simulink library "HDL_ieee_8021513"  (R2024a)
settings: Solver=FixedStepDiscrete  StartTime=0.0  StopTime=10.0  RelTol=1e-3
undefined symbols (not defined in the file): Add, axiWidth, CONST, fs, peakDetectorThreshold, peakDetectorWindow, QAM, Shift
libraries: hdlsllib x199, $bdroot x91, whdlutilities x34, whdledac x9, simulink x8, whdlmod x6, dspsigops x5, dsphdlfiltering2 x4, embreciprocals x3, dsphdlsigops2 x2, commhdlcrc x2, dspstat3 x2
(part 2 of 6)

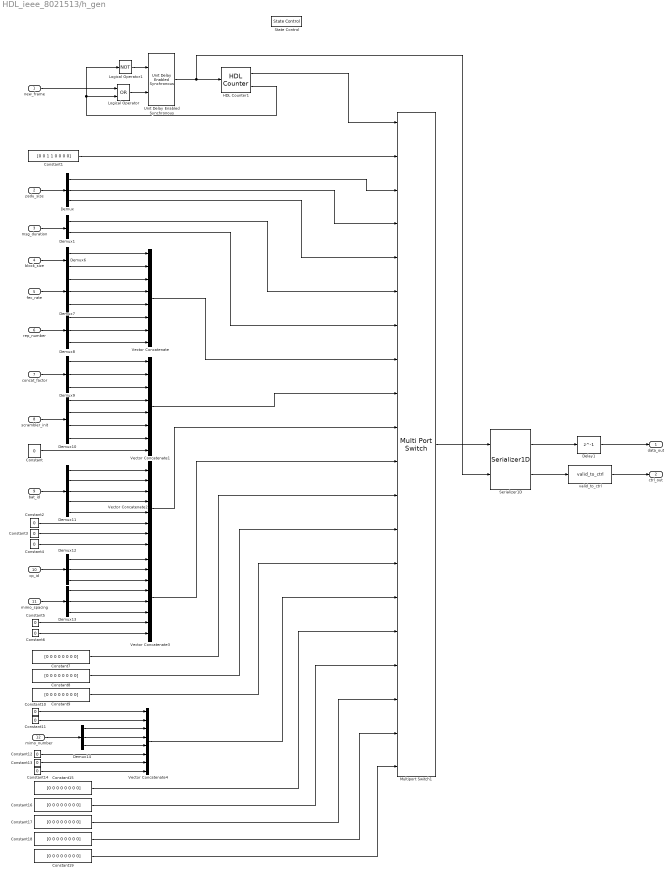
== system HDL_ieee_8021513/h_gen ==
  new_frame : Inport
  psdu_size : Inport  Port=2
  msg_duration : Inport  Port=3
  block_size : Inport  Port=4
  fec_rate : Inport  Port=5
  rep_number : Inport  Port=6
  concat_factor : Inport  Port=7
  scrambler_init : Inport  Port=8
  bat_id : Inport  Port=9
  cp_id : Inport  Port=10
  mimo_spacing : Inport  Port=11
  mimo_number : Inport  Port=12
  Constant{,2..6,10..14} (11 alike) : Constant  Value=0  OutDataTypeStr=boolean  SampleTime=-1
  Constant1 : Constant  Value=[0 0 1 1 0 0 0 0]  VectorParams1D=off  OutDataTypeStr=boolean  SampleTime=-1
  Constant{7..9,15..19} (8 alike) : Constant  Value=[0 0 0 0 0 0 0 0]  VectorParams1D=off  OutDataTypeStr=boolean  SampleTime=-1
  Delay1 : Delay  DelayLength=1  InitialCondition=0  UseCircularBuffer=on
  Demux{,7..9,12..14} (7 alike) : Demux  Outputs=3
  Demux1 : Demux  Outputs=2
  Demux10 : Demux
  Demux11 : Demux  Outputs=5
  Demux6 : Demux  Outputs=2
  HDL Counter1 : hdlsllib/Sources/HDL Counter  CountType=Count limited  CountInit=0  CountStep=1  CountMax=18  CountFromType=Initial value  CountFrom=0  CountResetPort=off  CountLoadPort=off  CountEnbPort=on  CountDirPort=off  CountHitOutputPort=on  CountDataType=Unsigned  CountWordLen=5  CountFracLen=0  CountSampTime=1
  Logical Operator : Logic  Operator=OR  IconShape=distinctive  AllPortsSameDT=off  OutDataTypeStr=boolean
  Logical Operator1 : Logic  Operator=NOT  IconShape=distinctive  AllPortsSameDT=off  OutDataTypeStr=boolean
  Multiport Switch1 : MultiPortSwitch  DataPortOrder=Zero-based contiguous  Inputs=19  zeroidx=on  OutDataTypeStr=Inherit: Same as first data input  SaturateOnIntegerOverflow=off
  Serializer1D : hdlsllib/HDL Operations/Serializer1D  Ratio=8  IdleCycles=0  validIn=on  startOut=off  validOut=on  inputDataDimensions=-1  inputSampleTime=-1  inputSignalType=auto
  State Control : StateControl  StateControl=Synchronous
  Unit Delay Enabled Synchronous : hdlsllib/Discrete/Unit Delay Enabled Synchronous  InitialCondition=0.0  SampleTime=-1
  Vector Concatenate{,1..4} (5 alike) : Concatenate  NumInputs=8  Mode=Multidimensional array  ConcatenateDimension=2
  valid_to_ctrl : $bdroot/valid_to_ctrl  SystemSampleTime=-1  VariantActivationTime=update diagram  AllowFlexibleInterface=on  Latency=0  AutoFrameSizeCalculation=off
  data_out : Outport  VectorParamsAs1DForOutWhenUnconnected=off
  ctrl_out : Outport  Port=2  VectorParamsAs1DForOutWhenUnconnected=off
  wires:
  mimo_number/1 -> Demux14/1
  msg_duration/1 -> Demux1/1
  rep_number/1 -> Demux8/1
  fec_rate/1 -> Demux7/1
  block_size/1 -> Demux6/1
  concat_factor/1 -> Demux9/1
  scrambler_init/1 -> Demux10/1
  Demux/2 -> Multiport Switch1/4
  Demux/3 -> Multiport Switch1/5
  Demux1/2 -> Multiport Switch1/7
  Constant1/1 -> Multiport Switch1/2
  Vector Concatenate/1 -> Multiport Switch1/8
  Constant/1 -> Vector Concatenate1/8
  bat_id/1 -> Demux11/1
  Constant2/1 -> Vector Concatenate2/6
  Constant3/1 -> Vector Concatenate2/7
  Constant4/1 -> Vector Concatenate2/8
  Constant5/1 -> Vector Concatenate3/7
  Constant6/1 -> Vector Concatenate3/8
  Constant10/1 -> Vector Concatenate4/1
  Constant11/1 -> Vector Concatenate4/2
  Constant12/1 -> Vector Concatenate4/6
  Constant13/1 -> Vector Concatenate4/7
  Constant14/1 -> Vector Concatenate4/8
  Vector Concatenate1/1 -> Multiport Switch1/9
  Vector Concatenate2/1 -> Multiport Switch1/10
  Vector Concatenate3/1 -> Multiport Switch1/11
  Constant7/1 -> Multiport Switch1/12
  Constant8/1 -> Multiport Switch1/13
  Constant9/1 -> Multiport Switch1/14
  Vector Concatenate4/1 -> Multiport Switch1/15
  Constant15/1 -> Multiport Switch1/16
  Constant16/1 -> Multiport Switch1/17
  Constant17/1 -> Multiport Switch1/18
  Constant18/1 -> Multiport Switch1/19
  Constant19/1 -> Multiport Switch1/20
  HDL Counter1/1 -> Multiport Switch1/1
  Multiport Switch1/1 -> Serializer1D/1
  Serializer1D/1 -> Delay1/1
  new_frame/1 -> Logical Operator/1
  HDL Counter1/2 -> Logical Operator/2, Logical Operator1/1
  Logical Operator/1 -> Unit Delay Enabled Synchronous/2
  Unit Delay Enabled Synchronous/1 -> Serializer1D/2, HDL Counter1/1
  Logical Operator1/1 -> Unit Delay Enabled Synchronous/1
  Delay1/1 -> data_out/1
  Serializer1D/2 -> valid_to_ctrl/1
  valid_to_ctrl/1 -> ctrl_out/1
  Demux6/1 -> Vector Concatenate/1
  Demux6/2 -> Vector Concatenate/2
  Demux7/1 -> Vector Concatenate/3
  Demux7/2 -> Vector Concatenate/4
  Demux7/3 -> Vector Concatenate/5
  Demux8/1 -> Vector Concatenate/6
  Demux8/2 -> Vector Concatenate/7
  Demux8/3 -> Vector Concatenate/8
  Demux9/1 -> Vector Concatenate1/1
  Demux9/2 -> Vector Concatenate1/2
  Demux9/3 -> Vector Concatenate1/3
  Demux10/1 -> Vector Concatenate1/4
  Demux10/2 -> Vector Concatenate1/5
  Demux10/3 -> Vector Concatenate1/6
  Demux10/4 -> Vector Concatenate1/7
  Demux11/1 -> Vector Concatenate2/1
  Demux11/2 -> Vector Concatenate2/2
  Demux11/3 -> Vector Concatenate2/3
  Demux11/4 -> Vector Concatenate2/4
  Demux11/5 -> Vector Concatenate2/5
  Demux12/1 -> Vector Concatenate3/1
  Demux12/2 -> Vector Concatenate3/2
  Demux12/3 -> Vector Concatenate3/3
  Demux13/1 -> Vector Concatenate3/4
  Demux13/2 -> Vector Concatenate3/5
  Demux13/3 -> Vector Concatenate3/6
  Demux14/1 -> Vector Concatenate4/3
  Demux14/2 -> Vector Concatenate4/4
  Demux14/3 -> Vector Concatenate4/5
  psdu_size/1 -> Demux/1
  cp_id/1 -> Demux12/1
  mimo_spacing/1 -> Demux13/1
  Demux/1 -> Multiport Switch1/3
  Demux1/1 -> Multiport Switch1/6

== system HDL_ieee_8021513/h_remove_repetition ==
  data_in : Inport
  start_in : Inport  Port=2
  HDL Counter : hdlsllib/Sources/HDL Counter  CountType=Count limited  CountInit=0  CountStep=1  CountMax=CONST.headerBitsPerFec-1  CountFromType=Initial value  CountFrom=0  CountResetPort=on  CountLoadPort=off  CountEnbPort=on  CountDirPort=off  CountHitOutputPort=on  CountDataType=Unsigned  CountWordLen=nextpow2(CONST.headerBitsPerFec)  CountFracLen=0  CountSampTime=1
  Logical Operator : Logic  Operator=OR  AllPortsSameDT=off  OutDataTypeStr=boolean
  Sample Control Bus Creator : whdlutilities/Sample Control Bus Creator
  State Control : StateControl  StateControl=Synchronous
  Switch : Switch  Criteria=u2 ~= 0  SaturateOnIntegerOverflow=off  InputSameDT=off
  Terminator : Terminator
  Unit Delay{,1..7} (8 alike) : UnitDelay  SampleTime=-1  HasFrameUpgradeWarning=on
  data_out : Outport
  ctrl_out : Outport  Port=2
  wires:
  Unit Delay7/1 -> Sample Control Bus Creator/3
  Unit Delay6/1 -> Sample Control Bus Creator/1
  Unit Delay5/1 -> data_out/1
  Switch/1 -> Unit Delay/1, HDL Counter/2, Unit Delay7/1
  Unit Delay3/1 -> HDL Counter/1, Unit Delay6/1  "rst"
  Unit Delay4/1 -> Unit Delay5/1  "data_in"
  Unit Delay2/1 -> Switch/1
  Unit Delay1/1 -> Switch/2
  Logical Operator/1 -> Unit Delay1/1
  HDL Counter/1 -> Terminator/1  "count"
  Unit Delay/1 -> Switch/3
  Sample Control Bus Creator/1 -> ctrl_out/1
  data_in/1 -> Unit Delay4/1
  HDL Counter/2 -> Sample Control Bus Creator/2, Logical Operator/2
  start_in/1 -> Unit Delay2/1, Logical Operator/1, Unit Delay3/1

== system HDL_ieee_8021513/h_repetition ==
  data_in : Inport
  ctrl_in : Inport  Port=2
  Bus Selector : BusSelector  OutputSignals=start,end,valid
  Delay{,1..4} (5 alike) : Delay  DelayLength=1  InitialCondition=0  UseCircularBuffer=on
  HDL Counter2 : hdlsllib/Sources/HDL Counter  CountType=Count limited  CountInit=CONST.headerBitsPerFec-2  CountStep=1  CountMax=CONST.headerBitsPerFec-1  CountFromType=Specify  CountFrom=0  CountResetPort=off  CountLoadPort=off  CountEnbPort=on  CountDirPort=off  CountHitOutputPort=off  CountDataType=Unsigned  CountWordLen=nextpow2(CONST.headerBitsPerOFDMSymbol)  CountFracLen=0  CountSampTime=1
  HDL Counter3 : hdlsllib/Sources/HDL Counter  CountType=Count limited  CountInit=0  CountStep=1  CountMax=CONST.headerBitsPerOFDMSymbol - CONST.headerBitsPerFec -1  CountFromType=Initial value  CountFrom=0  CountResetPort=off  CountLoadPort=off  CountEnbPort=on  CountDirPort=off  CountHitOutputPort=on  CountDataType=Unsigned  CountWordLen=nextpow2(CONST.headerBitsPerOFDMSymbol)  CountFracLen=0  CountSampTime=1
  Logical Operator : Logic  Operator=NOT  IconShape=distinctive  AllPortsSameDT=off  OutDataTypeStr=boolean
  Logical Operator1 : Logic  Operator=OR  IconShape=distinctive  AllPortsSameDT=off  OutDataTypeStr=boolean
  Logical Operator2 : Logic  Operator=NOT  IconShape=distinctive  AllPortsSameDT=off  OutDataTypeStr=boolean
  NOT : Logic  Operator=NOT  IconShape=distinctive  AllPortsSameDT=off  OutDataTypeStr=boolean
  Sample Control Bus Creator : whdlutilities/Sample Control Bus Creator
  Simple Dual Port RAM : hdlsllib/HDL RAMs/Simple Dual Port RAM  ram_size=nextpow2(CONST.headerBitsPerOFDMSymbol)
  State Control : StateControl  StateControl=Synchronous
  Switch : Switch  Criteria=u2 ~= 0  SaturateOnIntegerOverflow=off  InputSameDT=off
  Switch1 : Switch  Criteria=u2 ~= 0  SaturateOnIntegerOverflow=off  InputSameDT=off
  Unit Delay Enabled Synchronous1 : hdlsllib/Discrete/Unit Delay Enabled Synchronous  InitialCondition=0.0  SampleTime=-1
  data_out : Outport  VectorParamsAs1DForOutWhenUnconnected=off
  ctrl_out : Outport  Port=2  VectorParamsAs1DForOutWhenUnconnected=off
  wires:
  Delay4/1 -> [end_out]
  Delay3/1 -> Switch1/1
  ctrl_in/1 -> Bus Selector/1
  Bus Selector/3 -> [valid], Delay3/1  "<valid>"
  Sample Control Bus Creator/1 -> ctrl_out/1
  Bus Selector/1 -> Delay/1  "<start>"
  Bus Selector/2 -> [end]  "<end>"
  Delay/1 -> Sample Control Bus Creator/1
  [end_out] -> Sample Control Bus Creator/2
  Switch1/1 -> Sample Control Bus Creator/3
  [valid] -> HDL Counter2/1  "addrB_valid"
  [valid] -> Simple Dual Port RAM/3
  HDL Counter2/1 -> Simple Dual Port RAM/2
  data_in/1 -> Delay1/1, Simple Dual Port RAM/1  "datain"
  HDL Counter3/1 -> Simple Dual Port RAM/4  "addrA"
  Unit Delay Enabled Synchronous1/1 -> HDL Counter3/1, Delay2/1
  [end] -> Logical Operator1/1
  Logical Operator1/1 -> Unit Delay Enabled Synchronous1/2
  HDL Counter3/2 -> Logical Operator1/2, NOT/1, Delay4/1
  NOT/1 -> Unit Delay Enabled Synchronous1/1
  Switch/1 -> data_out/1
  Delay2/1 -> Logical Operator2/1, Switch1/3, Logical Operator/1
  Simple Dual Port RAM/1 -> Switch/3
  Delay1/1 -> Switch/1
  Logical Operator/1 -> Switch1/2
  Logical Operator2/1 -> Switch/2

== system HDL_ieee_8021513/h_rx_full ==
  data_in : Inport
  start_in : Inport  Port=2
  ldpc_in : Inport  Port=3
  ldpc_ctrl_in : Inport  Port=4
  Delay{2..5} (4 alike) : Delay  DelayLength=1  InitialCondition=0  UseCircularBuffer=on
  Rate Transition : RateTransition  OutPortSampleTimeOpt=Multiple of input port sample time  OutPortSampleTimeMultiple=8
  State Control : StateControl  StateControl=Synchronous
  h_crc_rx : $bdroot/h_crc_rx  SystemSampleTime=-1  VariantActivationTime=update diagram  AllowFlexibleInterface=on  Latency=0  AutoFrameSizeCalculation=off
  h_remove_repetition : $bdroot/h_remove_repetition  SystemSampleTime=-1  VariantActivationTime=update diagram  AllowFlexibleInterface=on  Latency=0  AutoFrameSizeCalculation=off
  h_scrambler : $bdroot/h_scrambler  SystemSampleTime=-1  VariantActivationTime=update diagram  AllowFlexibleInterface=on  Latency=0  AutoFrameSizeCalculation=off
      settings: LibrarySourceBlock=|
      | hdlsllib/Ports &
      | Subsystems/Subsystem
  h_separate : $bdroot/h_separate  SystemSampleTime=-1  VariantActivationTime=update diagram  AllowFlexibleInterface=on  Latency=0  AutoFrameSizeCalculation=off
  psdu_size : Outport
  msg_duration : Outport  Port=2
  block_size : Outport  Port=3
  fec_rate : Outport  Port=4
  rep_number : Outport  Port=5
  concat_factor : Outport  Port=6
  scrambler_init : Outport  Port=7
  bat_id : Outport  Port=8
  cp_id : Outport  Port=9
  mimo_spacing : Outport  Port=10
  mimo_number : Outport  Port=11
  end : Outport  Port=12
  err : Outport  Port=13
  ldpc_out : Outport  Port=14  VectorParamsAs1DForOutWhenUnconnected=off
  ldpc_ctrl_out : Outport  Port=15  VectorParamsAs1DForOutWhenUnconnected=off
  wires:
  Delay5/1 -> end/1
  Delay4/1 -> err/1
  Delay3/1 -> h_scrambler/2
  Delay2/1 -> h_scrambler/1
  h_remove_repetition/1 -> ldpc_out/1
  h_remove_repetition/2 -> ldpc_ctrl_out/1
  Rate Transition/1 -> Delay4/1
  h_separate/4 -> fec_rate/1
  h_separate/1 -> psdu_size/1
  ldpc_ctrl_in/1 -> Delay3/1
  h_crc_rx/2 -> h_separate/2
  h_scrambler/2 -> h_crc_rx/2
  h_separate/7 -> scrambler_init/1
  h_scrambler/1 -> h_crc_rx/1
  h_separate/5 -> rep_number/1
  h_separate/11 -> mimo_number/1
  h_crc_rx/1 -> h_separate/1
  h_separate/9 -> cp_id/1
  h_crc_rx/3 -> Rate Transition/1
  ldpc_in/1 -> Delay2/1
  h_separate/8 -> bat_id/1
  h_separate/2 -> msg_duration/1
  h_separate/10 -> mimo_spacing/1
  h_separate/6 -> concat_factor/1
  h_separate/12 -> Delay5/1
  h_separate/3 -> block_size/1
  data_in/1 -> h_remove_repetition/1
  start_in/1 -> h_remove_repetition/2

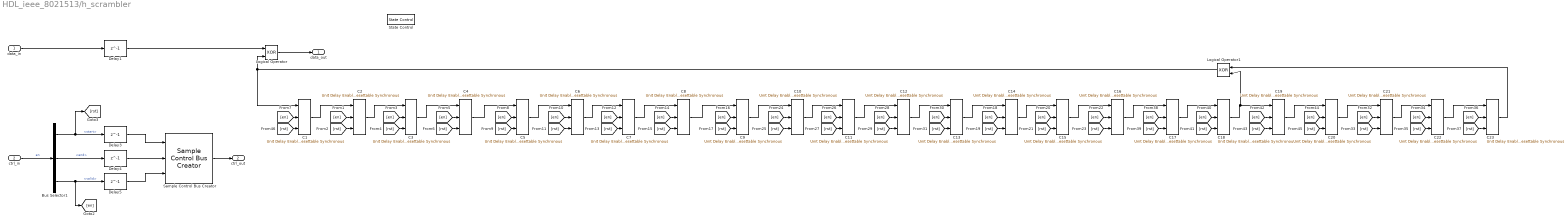
== system HDL_ieee_8021513/h_scrambler ==
  data_in : Inport
  ctrl_in : Inport  Port=2
  Bus Selector1 : BusSelector  OutputSignals=start,end,valid
  C{1,3,5,7,9,11,13,15,17,19,21,23} (12 alike) : hdlsllib/Discrete/Unit Delay Enabled Resettable Synchronous  InitialCondition=0  SampleTime=-1
  C{2,4,6,8,10,12,14,16,18,20,22} (11 alike) : hdlsllib/Discrete/Unit Delay Enabled Resettable Synchronous  InitialCondition=1  SampleTime=-1
  Delay{1,3..5} (4 alike) : Delay  DelayLength=1  InitialCondition=0  UseCircularBuffer=on
  Logical Operator : Logic  Operator=XOR  IconShape=distinctive  AllPortsSameDT=off  OutDataTypeStr=boolean
  Logical Operator1 : Logic  Operator=XOR  IconShape=distinctive  AllPortsSameDT=off  OutDataTypeStr=boolean
  Sample Control Bus Creator : whdlutilities/Sample Control Bus Creator
  State Control : StateControl  StateControl=Synchronous
  data_out : Outport
  ctrl_out : Outport  Port=2  VectorParamsAs1DForOutWhenUnconnected=off
  wires:
  Sample Control Bus Creator/1 -> ctrl_out/1
  Delay5/1 -> Sample Control Bus Creator/3
  Delay4/1 -> Sample Control Bus Creator/2
  Delay3/1 -> Sample Control Bus Creator/1
  Bus Selector1/3 -> Delay5/1, [en]  "<valid>"
  Bus Selector1/2 -> Delay4/1  "<end>"
  Bus Selector1/1 -> Delay3/1, [rst]  "<start>"
  C23/1 -> Logical Operator1/1
  [rst] -> C22/3
  C19/1 -> C20/1
  [en] -> C20/2
  [en] -> C21/2
  C21/1 -> C22/1
  [rst] -> C18/3
  [en] -> C17/2
  [rst] -> C19/3
  [rst] -> C21/3
  C17/1 -> C18/1
  C22/1 -> C23/1
  [en] -> C19/2
  [en] -> C18/2
  [en] -> C23/2
  [rst] -> C20/3
  [en] -> C22/2
  C16/1 -> C17/1
  [rst] -> C23/3
  [rst] -> C17/3
  C8/1 -> C9/1
  [rst] -> C15/3
  [en] -> C15/2
  [en] -> C14/2
  [rst] -> C16/3
  [en] -> C12/2
  [rst] -> C14/3
  C13/1 -> C14/1
  C11/1 -> C12/1
  [rst] -> C9/3
  [en] -> C10/2
  [en] -> C9/2
  C14/1 -> C15/1
  [en] -> C11/2
  [rst] -> C13/3
  C10/1 -> C11/1
  [rst] -> C10/3
  C12/1 -> C13/1
  [en] -> C13/2
  [rst] -> C11/3
  [en] -> C16/2
  [rst] -> C12/3
  C9/1 -> C10/1
  C15/1 -> C16/1
  [rst] -> C5/3
  [en] -> C6/2
  C6/1 -> C7/1
  [en] -> C8/2
  [rst] -> C6/3
  C5/1 -> C6/1
  [rst] -> C7/3
  C7/1 -> C8/1
  [rst] -> C8/3
  [en] -> C7/2
  [en] -> C5/2
  Delay1/1 -> Logical Operator/1
  data_in/1 -> Delay1/1
  ctrl_in/1 -> Bus Selector1/1  "en"
  Logical Operator/1 -> data_out/1
  [rst] -> C3/3
  [en] -> C3/2
  Logical Operator1/1 -> Logical Operator/2, C1/1
  [rst] -> C2/3
  C1/1 -> C2/1
  C3/1 -> C4/1
  [en] -> C1/2
  [rst] -> C1/3
  C4/1 -> C5/1
  [en] -> C4/2
  C2/1 -> C3/1
  [rst] -> C4/3
  [en] -> C2/2
  C20/1 -> C21/1
  C18/1 -> Logical Operator1/2, C19/1

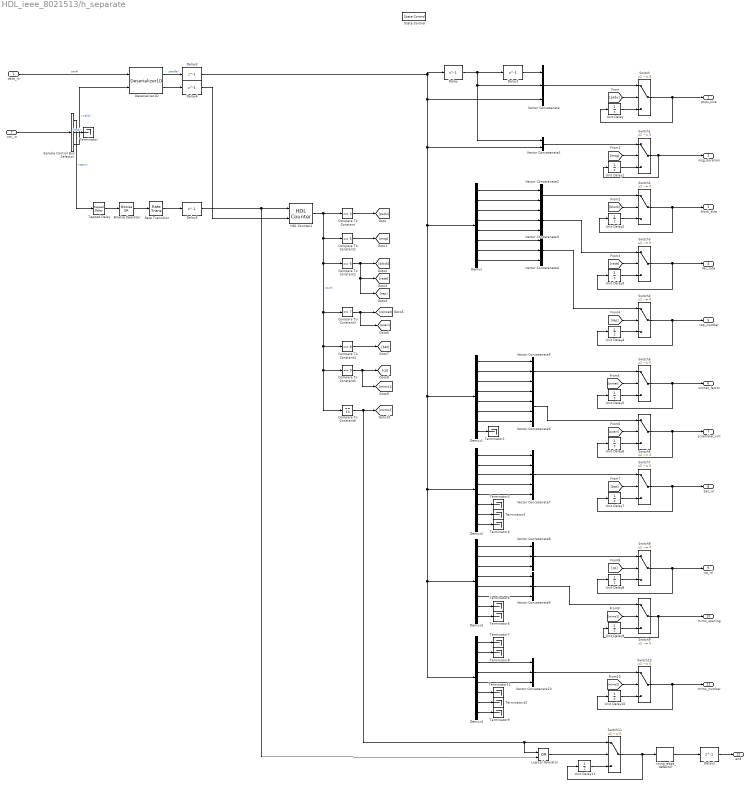
== system HDL_ieee_8021513/h_separate ==
  data_in : Inport
  ctrl_in : Inport  Port=2
  Bitwise Operator : simulink/Logic and Bit Operations/Bitwise Operator  logicop=OR  UseBitMask=off  BitMask=bin2dec('11011001')  BitMaskRealWorld=Stored Integer
      settings: LibrarySourceBlock=|
      | hdlsllib/Logic and Bit
      | Operations/Bitwise
      | Operator
  Compare To Constant : hdlsllib/Logic and Bit Operations/Compare To Constant  relop===  const=3  OutDataTypeStr=boolean
  Compare To Constant1 : hdlsllib/Logic and Bit Operations/Compare To Constant  relop===  const=5  OutDataTypeStr=boolean
  Compare To Constant2 : hdlsllib/Logic and Bit Operations/Compare To Constant  relop===  const=6  OutDataTypeStr=boolean
  Compare To Constant3 : hdlsllib/Logic and Bit Operations/Compare To Constant  relop===  const=7  OutDataTypeStr=boolean
  Compare To Constant4 : hdlsllib/Logic and Bit Operations/Compare To Constant  relop===  const=8  OutDataTypeStr=boolean
  Compare To Constant5 : hdlsllib/Logic and Bit Operations/Compare To Constant  relop===  const=9  OutDataTypeStr=boolean
  Compare To Constant6 : hdlsllib/Logic and Bit Operations/Compare To Constant  relop===  const=13  OutDataTypeStr=boolean
  Delay{,1..5} (6 alike) : Delay  DelayLength=1  InitialCondition=0  UseCircularBuffer=on
  Demux{,1..4} (5 alike) : Demux  Outputs=8
  Deserializer1D : hdlsllib/HDL Operations/Deserializer1D  Ratio=8  IdleCycles=0  InitialCondition=0  startIn=off  validIn=on  validOut=on  inputDataDimensions=-1  inputSampleTime=-1  inputSignalType=auto
  HDL Counter1 : hdlsllib/Sources/HDL Counter  CountType=Free running  CountInit=0  CountStep=1  CountMax=25  CountFromType=Initial value  CountFrom=0  CountResetPort=on  CountLoadPort=off  CountEnbPort=on  CountDirPort=off  CountHitOutputPort=off  CountDataType=Unsigned  CountWordLen=5  CountFracLen=0  CountSampTime=1
  Logical Operator : Logic  Operator=OR  IconShape=distinctive  AllPortsSameDT=off  OutDataTypeStr=boolean
  Rate Transition : RateTransition  OutPortSampleTimeOpt=Multiple of input port sample time  OutPortSampleTimeMultiple=8
  Sample Control Bus Selector : whdlutilities/Sample Control Bus Selector  OutputSignals=start,end,valid
  State Control : StateControl  StateControl=Synchronous
  Switch{,1..11} (12 alike) : Switch  Criteria=u2 ~= 0  SaturateOnIntegerOverflow=off  InputSameDT=off
  Tapped Delay : simulink/Discrete/Tapped Delay  vinit=0.0  samptime=-1  NumDelays=8  DelayOrder=Oldest  includeCurrent=off
      settings: LibrarySourceBlock=hdlsllib/Discrete/Tapped Delay
  Terminator{,1..11} (12 alike) : Terminator
  Unit Delay{,1..11} (12 alike) : UnitDelay  SampleTime=-1  HasFrameUpgradeWarning=on
  Vector Concatenate{,3..5,8..10} (7 alike) : Concatenate  NumInputs=3
  Vector Concatenate1 : Concatenate
  Vector Concatenate2 : Concatenate
  Vector Concatenate6 : Concatenate  NumInputs=4
  Vector Concatenate7 : Concatenate  NumInputs=5
  rising_edge_detector : $bdroot/rising_edge_detector  SystemSampleTime=-1  VariantActivationTime=update diagram  AllowFlexibleInterface=on  Latency=0  AutoFrameSizeCalculation=off
  psdu_size : Outport
  msg_duration : Outport  Port=2
  block_size : Outport  Port=3
  fec_rate : Outport  Port=4
  rep_number : Outport  Port=5
  concat_factor : Outport  Port=6
  scrambler_init : Outport  Port=7
  bat_id : Outport  Port=8
  cp_id : Outport  Port=9
  mimo_spacing : Outport  Port=10
  mimo_number : Outport  Port=11
  end : Outport  Port=12  VectorParamsAs1DForOutWhenUnconnected=off
  wires:
  Delay5/1 -> HDL Counter1/1, Logical Operator/2
  Delay4/1 -> HDL Counter1/2
  Delay3/1 -> Vector Concatenate/3, Vector Concatenate1/2, Demux/1, Demux1/1, Demux2/1, Demux3/1, Demux4/1, Delay/1
  rising_edge_detector/1 -> Delay2/1
  Bitwise Operator/1 -> Rate Transition/1
  Tapped Delay/1 -> Bitwise Operator/1
  Delay2/1 -> end/1
  Logical Operator/1 -> Switch11/2
  Compare To Constant6/1 -> [mimo2], Switch11/1, Logical Operator/1
  Unit Delay11/1 -> Switch11/3
  Switch11/1 -> rising_edge_detector/1, Unit Delay11/1
  Vector Concatenate10/1 -> Switch10/1
  Demux4/5 -> Vector Concatenate10/3
  Demux4/4 -> Vector Concatenate10/2
  Demux4/3 -> Vector Concatenate10/1
  Demux4/6 -> Terminator11/1
  Demux4/7 -> Terminator10/1
  Demux4/8 -> Terminator9/1
  Demux4/2 -> Terminator8/1
  Demux4/1 -> Terminator7/1
  Vector Concatenate9/1 -> Switch9/1
  Vector Concatenate8/1 -> Switch8/1
  Demux3/3 -> Vector Concatenate8/3
  Demux3/2 -> Vector Concatenate8/2
  Demux3/1 -> Vector Concatenate8/1
  Demux3/6 -> Vector Concatenate9/3
  Demux3/5 -> Vector Concatenate9/2
  Demux3/4 -> Vector Concatenate9/1
  Demux3/7 -> Terminator6/1
  Demux3/8 -> Terminator5/1
  Vector Concatenate7/1 -> Switch7/1
  Demux2/5 -> Vector Concatenate7/5
  Demux2/4 -> Vector Concatenate7/4
  Demux2/3 -> Vector Concatenate7/3
  Demux2/2 -> Vector Concatenate7/2
  Demux2/1 -> Vector Concatenate7/1
  Demux2/8 -> Terminator4/1
  Demux2/7 -> Terminator3/1
  Demux2/6 -> Terminator2/1
  Vector Concatenate6/1 -> Switch6/1
  Demux1/8 -> Terminator1/1
  Demux1/7 -> Vector Concatenate6/4
  Demux1/6 -> Vector Concatenate6/3
  Demux1/5 -> Vector Concatenate6/2
  Demux1/4 -> Vector Concatenate6/1
  Vector Concatenate5/1 -> Switch5/1
  Demux1/3 -> Vector Concatenate5/3
  Demux1/2 -> Vector Concatenate5/2
  Demux1/1 -> Vector Concatenate5/1
  Vector Concatenate4/1 -> Switch4/1
  Demux/8 -> Vector Concatenate4/3
  Demux/7 -> Vector Concatenate4/2
  Demux/6 -> Vector Concatenate4/1
  Vector Concatenate3/1 -> Switch3/1
  Demux/5 -> Vector Concatenate3/3
  Demux/4 -> Vector Concatenate3/2
  Demux/3 -> Vector Concatenate3/1
  Vector Concatenate2/1 -> Switch2/1
  Demux/2 -> Vector Concatenate2/2
  Demux/1 -> Vector Concatenate2/1
  Sample Control Bus Selector/2 -> Terminator/1  "<end>"
  Vector Concatenate1/1 -> Switch1/1
  [mimo2] -> Switch10/2
  Switch10/1 -> Unit Delay10/1, mimo_number/1
  Unit Delay10/1 -> Switch10/3
  [mimo1] -> Switch9/2
  Switch9/1 -> Unit Delay9/1, mimo_spacing/1
  Unit Delay9/1 -> Switch9/3
  [cp] -> Switch8/2
  Switch8/1 -> Unit Delay8/1, cp_id/1
  Unit Delay8/1 -> Switch8/3
  [bat] -> Switch7/2
  Switch7/1 -> Unit Delay7/1, bat_id/1
  Unit Delay7/1 -> Switch7/3
  [scram] -> Switch6/2
  Switch6/1 -> Unit Delay6/1, scrambler_init/1
  Unit Delay6/1 -> Switch6/3
  [concat] -> Switch5/2
  Switch5/1 -> Unit Delay5/1, concat_factor/1
  Unit Delay5/1 -> Switch5/3
  [rep] -> Switch4/2
  Switch4/1 -> Unit Delay4/1, rep_number/1
  Unit Delay4/1 -> Switch4/3
  [rate] -> Switch3/2
  Switch3/1 -> Unit Delay3/1, fec_rate/1
  Unit Delay3/1 -> Switch3/3
  [block] -> Switch2/2
  Switch2/1 -> Unit Delay2/1, block_size/1
  Unit Delay2/1 -> Switch2/3
  Switch1/1 -> Unit Delay1/1, msg_duration/1
  Unit Delay1/1 -> Switch1/3
  [msg] -> Switch1/2
  [psdu] -> Switch/2
  Compare To Constant5/1 -> [cp], [mimo1]
  Compare To Constant4/1 -> [bat]
  Compare To Constant3/1 -> [concat], [scram]
  Compare To Constant2/1 -> [rep], [rate], [block]
  Compare To Constant1/1 -> [msg]
  Compare To Constant/1 -> [psdu]
  HDL Counter1/1 -> Compare To Constant/1, Compare To Constant1/1, Compare To Constant2/1, Compare To Constant3/1, Compare To Constant4/1, Compare To Constant5/1, Compare To Constant6/1  "count"
  Rate Transition/1 -> Delay5/1
  Deserializer1D/2 -> Delay4/1
  Unit Delay/1 -> Switch/3
  Switch/1 -> psdu_size/1, Unit Delay/1
  Vector Concatenate/1 -> Switch/1
  Delay1/1 -> Vector Concatenate/1
  Delay/1 -> Delay1/1, Vector Concatenate/2, Vector Concatenate1/1
  Deserializer1D/1 -> Delay3/1  "parallel"
  data_in/1 -> Deserializer1D/1  "serial"
  Sample Control Bus Selector/1 -> Tapped Delay/1  "<start>"
  Sample Control Bus Selector/3 -> Deserializer1D/2  "<valid>"
  ctrl_in/1 -> Sample Control Bus Selector/1

== system HDL_ieee_8021513/header_fec ==
  data_in : Inport
  ctrl_in : Inport  Port=2
  Delay{,1..3} (4 alike) : Delay  DelayLength=1  InitialCondition=0  UseCircularBuffer=on
  Hc_12H_B14 : whdledac/LDPC Encoder  ParityCheckMatrix=CONST.Hc_12H  BlockSize=14  SimulateUsing=Code generation
  State Control : StateControl  StateControl=Synchronous
  Terminator : Terminator
  data_out : Outport
  ctrl_out : Outport  Port=2
  wires:
  Delay3/1 -> Hc_12H_B14/1
  Delay2/1 -> Hc_12H_B14/2
  Delay1/1 -> data_out/1
  Delay/1 -> ctrl_out/1
  ctrl_in/1 -> Delay2/1
  data_in/1 -> Delay3/1
  Hc_12H_B14/2 -> Delay/1
  Hc_12H_B14/1 -> Delay1/1
  Hc_12H_B14/3 -> Terminator/1

== system HDL_ieee_8021513/header_full ==
  new_frame : Inport
  psdu_size : Inport  Port=2
  msg_duration : Inport  Port=3
  block_size : Inport  Port=4
  fec_rate : Inport  Port=5
  rep_number : Inport  Port=6
  concat_factor : Inport  Port=7
  scrambler_init : Inport  Port=8
  bat_id : Inport  Port=9
  cp_id : Inport  Port=10
  mimo_spacing : Inport  Port=11
  mimo_number : Inport  Port=12
  State Control : StateControl  StateControl=Synchronous
  h_crc : $bdroot/h_crc  SystemSampleTime=-1  VariantActivationTime=update diagram  AllowFlexibleInterface=on  Latency=0  AutoFrameSizeCalculation=off
  h_gen : $bdroot/h_gen  SystemSampleTime=-1  VariantActivationTime=update diagram  AllowFlexibleInterface=on  Latency=0  AutoFrameSizeCalculation=off
  h_repetition : $bdroot/h_repetition  SystemSampleTime=-1  VariantActivationTime=update diagram  AllowFlexibleInterface=on  Latency=0  AutoFrameSizeCalculation=off
  h_scrambler : $bdroot/h_scrambler  SystemSampleTime=-1  VariantActivationTime=update diagram  AllowFlexibleInterface=on  Latency=0  AutoFrameSizeCalculation=off
      settings: LibrarySourceBlock=|
      | hdlsllib/Ports &
      | Subsystems/Subsystem
  header_fec : $bdroot/header_fec  SystemSampleTime=-1  VariantActivationTime=update diagram  AllowFlexibleInterface=on  Latency=0  AutoFrameSizeCalculation=off
  header : Outport  VectorParamsAs1DForOutWhenUnconnected=off
  ctrl_out : Outport  Port=2  VectorParamsAs1DForOutWhenUnconnected=off
  wires:
  h_scrambler/1 -> header_fec/1
  h_scrambler/2 -> header_fec/2
  header_fec/1 -> h_repetition/1  "dataOut"
  header_fec/2 -> h_repetition/2
  h_crc/2 -> h_scrambler/2
  h_crc/1 -> h_scrambler/1
  h_gen/2 -> h_crc/2
  h_gen/1 -> h_crc/1
  h_repetition/2 -> ctrl_out/1
  h_repetition/1 -> header/1
  new_frame/1 -> h_gen/1
  psdu_size/1 -> h_gen/2
  msg_duration/1 -> h_gen/3
  block_size/1 -> h_gen/4
  fec_rate/1 -> h_gen/5
  rep_number/1 -> h_gen/6
  concat_factor/1 -> h_gen/7
  scrambler_init/1 -> h_gen/8
  bat_id/1 -> h_gen/9
  cp_id/1 -> h_gen/10
  mimo_spacing/1 -> h_gen/11
  mimo_number/1 -> h_gen/12

== system HDL_ieee_8021513/interpolator ==
  data_in : Inport
  valid_in : Inport  Port=2
  Delay{,4,6..11,14..15,18} (11 alike) : Delay  DelayLength=1  InitialCondition=0  UseCircularBuffer=on
  Delay1 : Delay  DelayLength=CONST.txInterpolatorDelay  InitialCondition=0  UseCircularBuffer=on
  Delay16 : Delay  DelayLength=CONST.txInterpolatorDelay*(CONST.txL-1)  InitialCondition=0  UseCircularBuffer=on
  Delay17 : Delay  DelayLength=CONST.txInterpolatorDelay*(CONST.txL-1)  InitialCondition=0  UseCircularBuffer=on
  Delay2 : Delay  InitialCondition=0  UseCircularBuffer=on
  Delay3 : Delay  DelayLength=CONST.txInterpolatorDelay  InitialCondition=0  UseCircularBuffer=on
  Delay5 : Delay  InitialCondition=0  UseCircularBuffer=on
  FIR Interpolator : dsphdlfiltering2/FIR Interpolator  Numerator=CONST.txInterpolatorFilter.Numerator  FilterStructure=Direct form systolic  InterpolationFactor=CONST.txL  NumCycles=CONST.txL  SimulateUsing=Code generation  roundingMode=Floor  overflowMode=off  CoefficientsDataTypeStr=CONST.txInterpolatorCoefficientsDataType  OutputDataTypeStr=CONST.txInterpolatorOutputDataType  ResetInputPort=off  HDLGlobalReset=on
  HDL Counter : hdlsllib/Sources/HDL Counter  CountType=Count limited  CountInit=0  CountStep=1  CountMax=CONST.txInterpolatorDelay*(CONST.txL-1)-1  CountFromType=Initial value  CountFrom=0  CountResetPort=on  CountLoadPort=off  CountEnbPort=on  CountDirPort=off  CountHitOutputPort=on  CountDataType=Unsigned  CountWordLen=8  CountFracLen=0  CountSampTime=1
  Logical Operator : Logic  Operator=OR  IconShape=distinctive  AllPortsSameDT=off  OutDataTypeStr=boolean
  Logical Operator1 : Logic  IconShape=distinctive  AllPortsSameDT=off  OutDataTypeStr=boolean
  Logical Operator2 : Logic  AllPortsSameDT=off  OutDataTypeStr=boolean
  Logical Operator3 : Logic  Operator=NOT  AllPortsSameDT=off  OutDataTypeStr=boolean
  Logical Operator4 : Logic  Operator=OR  AllPortsSameDT=off  OutDataTypeStr=boolean
  State Control : StateControl  StateControl=Synchronous
  Switch : Switch  Criteria=u2 ~= 0  SaturateOnIntegerOverflow=off  InputSameDT=off
  Terminator : Terminator
  Terminator1 : Terminator
  Unit Delay : UnitDelay  SampleTime=-1  HasFrameUpgradeWarning=on
  Upsample : dspsigops/Upsample  FactorSource=Dialog parameter  N=CONST.txL  Nmax=16  phase=0  RateOptions=Allow multirate processing  ic=0  mode=Unused parameter value
      settings: LibrarySourceBlock=dsphdlsupportsigops/Upsample
  Upsample1 : dspsigops/Upsample  FactorSource=Dialog parameter  N=CONST.txL  Nmax=16  phase=0  RateOptions=Allow multirate processing  ic=0  mode=Unused parameter value
      settings: LibrarySourceBlock=dsphdlsupportsigops/Upsample
  falling_edge_detector : $bdroot/falling_edge_detector  SystemSampleTime=-1  VariantActivationTime=update diagram  AllowFlexibleInterface=on  Latency=0  AutoFrameSizeCalculation=off
  data_out : Outport  VectorParamsAs1DForOutWhenUnconnected=off
  valid_out : Outport  Port=2  VectorParamsAs1DForOutWhenUnconnected=off
  wires:
  Delay18/1 -> Logical Operator3/1
  Logical Operator3/1 -> Logical Operator2/2
  Delay7/1 -> Logical Operator4/2
  Logical Operator4/1 -> Switch/2
  Delay15/1 -> Delay16/1
  Delay14/1 -> Delay15/1
  Delay17/1 -> Delay4/1
  Delay16/1 -> Logical Operator2/1
  Delay10/1 -> HDL Counter/1, Switch/1, Logical Operator4/1
  Switch/1 -> Unit Delay/1, HDL Counter/2, Delay18/1  "count_enable"
  Unit Delay/1 -> Switch/3
  HDL Counter/1 -> Terminator/1  "count"
  HDL Counter/2 -> Delay7/1
  Logical Operator2/1 -> Delay/1
  Delay11/1 -> Delay17/1
  Delay9/1 -> Delay6/1
  Delay8/1 -> Delay14/1, falling_edge_detector/1
  Delay6/1 -> Delay11/1
  falling_edge_detector/1 -> Delay10/1  "b"
  Delay5/1 -> Upsample/1
  Delay2/1 -> Upsample1/1
  data_in/1 -> Delay5/1
  FIR Interpolator/1 -> Delay9/1
  Upsample1/1 -> FIR Interpolator/2
  valid_in/1 -> Delay3/1, Logical Operator/1
  Delay/1 -> valid_out/1
  FIR Interpolator/3 -> Terminator1/1
  Delay1/1 -> Logical Operator1/2
  Delay3/1 -> Logical Operator/2
  Logical Operator/1 -> Delay2/1
  Upsample/1 -> FIR Interpolator/1
  Logical Operator1/1 -> Delay8/1
  Delay4/1 -> data_out/1
  FIR Interpolator/2 -> Delay1/1, Logical Operator1/1

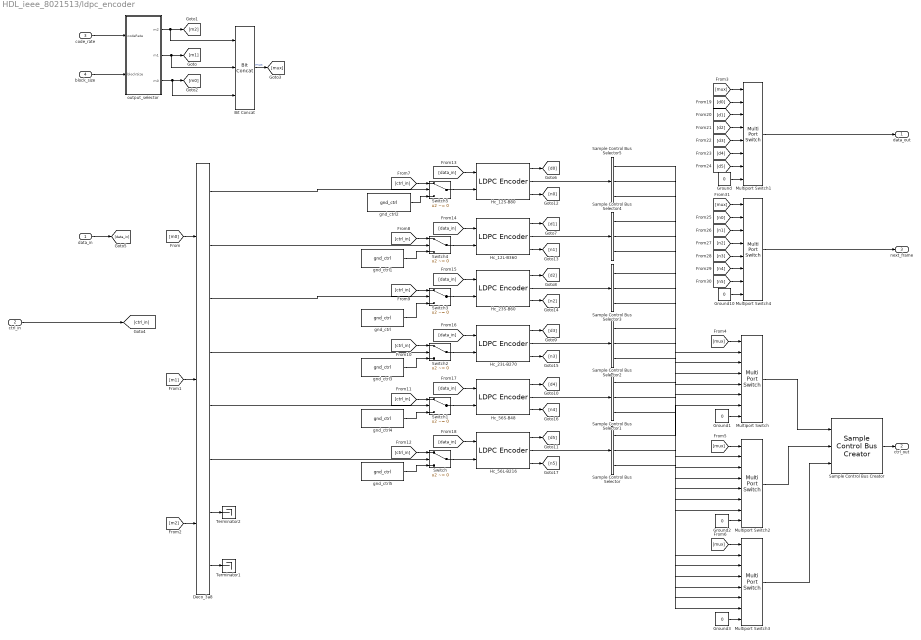
== system HDL_ieee_8021513/ldpc_encoder ==
  data_in : Inport
  ctrl_in : Inport  Port=2
  code_rate : Inport  Port=3
  block_size : Inport  Port=4
  Bit Concat : hdlsllib/Logic and Bit Operations/Bit Concat  numInputs=3
  Deco_3a8 : $bdroot/Deco_3a8  SystemSampleTime=-1  VariantActivationTime=update diagram  AllowFlexibleInterface=on  Latency=0  AutoFrameSizeCalculation=off
  Ground{,1..3,10} (5 alike) : Constant  Value=0  OutDataTypeStr=Inherit: Inherit via back propagation  SampleTime=-1
  Hc_12L-B360 : whdledac/LDPC Encoder  ParityCheckMatrix=CONST.Hc_12L  BlockSize=360  SimulateUsing=Code generation
  Hc_12S-B80 : whdledac/LDPC Encoder  ParityCheckMatrix=CONST.Hc_12S  BlockSize=80  SimulateUsing=Code generation
  Hc_23L-B270 : whdledac/LDPC Encoder  ParityCheckMatrix=CONST.Hc_23L  BlockSize=270  SimulateUsing=Code generation
  Hc_23S-B60 : whdledac/LDPC Encoder  ParityCheckMatrix=CONST.Hc_23S  BlockSize=60  SimulateUsing=Code generation
  Hc_56L-B216 : whdledac/LDPC Encoder  ParityCheckMatrix=CONST.Hc_56L  BlockSize=216  SimulateUsing=Code generation
  Hc_56S-B48 : whdledac/LDPC Encoder  ParityCheckMatrix=CONST.Hc_56S  BlockSize=48  SimulateUsing=Code generation
  Multiport Switch{,1..4} (5 alike) : MultiPortSwitch  DataPortOrder=Zero-based contiguous  Inputs=6  DataPortForDefault=Additional data port  DiagnosticForDefault=None  zeroidx=on  SaturateOnIntegerOverflow=off  InputSameDT=off
  Sample Control Bus Creator : whdlutilities/Sample Control Bus Creator
  Sample Control Bus Selector{,1..5} (6 alike) : whdlutilities/Sample Control Bus Selector  OutputSignals=start,end,valid
  Switch{,1..5} (6 alike) : Switch  Criteria=u2 ~= 0  SaturateOnIntegerOverflow=off  InputSameDT=off  OutDataTypeStr=Inherit: Same as first input
  Terminator1 : Terminator
  Terminator2 : Terminator
  gnd_ctrl{,1..5} (6 alike) : $bdroot/gnd_ctrl  SystemSampleTime=-1  VariantActivationTime=update diagram  AllowFlexibleInterface=on  Latency=0  AutoFrameSizeCalculation=off
  output_selector : Subsystem
  data_out : Outport
  ctrl_out : Outport  Port=2
  next_frame : Outport  Port=3
  wires:
  Multiport Switch1/1 -> data_out/1
  Switch/1 -> Hc_56L-B216/2
  Deco_3a8/8 -> Terminator1/1
  Deco_3a8/7 -> Terminator2/1
  Deco_3a8/6 -> Switch/2
  Switch5/1 -> Hc_12S-B80/2
  Switch4/1 -> Hc_12L-B360/2
  Switch3/1 -> Hc_23S-B60/2
  Switch2/1 -> Hc_23L-B270/2
  Switch1/1 -> Hc_56S-B48/2
  Deco_3a8/1 -> Switch5/2
  Deco_3a8/2 -> Switch4/2
  Deco_3a8/3 -> Switch3/2
  Deco_3a8/4 -> Switch2/2
  Deco_3a8/5 -> Switch1/2
  Hc_12L-B360/3 -> [n1]
  Hc_12S-B80/3 -> [n0]
  Hc_23S-B60/3 -> [n2]
  Hc_23L-B270/3 -> [n3]
  Hc_56S-B48/3 -> [n4]
  Hc_56L-B216/3 -> [n5]
  gnd_ctrl/1 -> Switch3/3
  Hc_56L-B216/2 -> Sample Control Bus Selector/1
  Sample Control Bus Selector/3 -> Multiport Switch3/7
  Sample Control Bus Selector/2 -> Multiport Switch2/7
  Sample Control Bus Selector/1 -> Multiport Switch/7
  Hc_56S-B48/2 -> Sample Control Bus Selector1/1
  Sample Control Bus Selector1/3 -> Multiport Switch3/6
  Sample Control Bus Selector1/2 -> Multiport Switch2/6
  Sample Control Bus Selector1/1 -> Multiport Switch/6
  Hc_23L-B270/2 -> Sample Control Bus Selector2/1
  Sample Control Bus Selector2/3 -> Multiport Switch3/5
  Sample Control Bus Selector2/2 -> Multiport Switch2/5
  Sample Control Bus Selector2/1 -> Multiport Switch/5
  Hc_23S-B60/2 -> Sample Control Bus Selector3/1
  Sample Control Bus Selector3/3 -> Multiport Switch3/4
  Sample Control Bus Selector3/2 -> Multiport Switch2/4
  Sample Control Bus Selector3/1 -> Multiport Switch/4
  Hc_12L-B360/2 -> Sample Control Bus Selector4/1
  Sample Control Bus Selector4/1 -> Multiport Switch/3
  Sample Control Bus Selector4/3 -> Multiport Switch3/3
  Sample Control Bus Selector4/2 -> Multiport Switch2/3
  Hc_12S-B80/2 -> Sample Control Bus Selector5/1
  Sample Control Bus Selector5/3 -> Multiport Switch3/2
  Sample Control Bus Selector5/2 -> Multiport Switch2/2
  Sample Control Bus Selector5/1 -> Multiport Switch/2
  Multiport Switch/1 -> Sample Control Bus Creator/1
  Multiport Switch2/1 -> Sample Control Bus Creator/2
  Multiport Switch3/1 -> Sample Control Bus Creator/3
  Sample Control Bus Creator/1 -> ctrl_out/1
  Ground/1 -> Multiport Switch1/8
  Ground1/1 -> Multiport Switch/8
  Ground2/1 -> Multiport Switch2/8
  Ground3/1 -> Multiport Switch3/8
  code_rate/1 -> output_selector/1(codeRate)
  block_size/1 -> output_selector/2(blockSize)
  output_selector/1(m2) -> Bit Concat/1, [m2]
  output_selector/3(m0) -> Bit Concat/3, [m0]
  output_selector/2(m1) -> Bit Concat/2, [m1]
  Bit Concat/1 -> [mux]  "mux"
  [m0] -> Deco_3a8/1
  [m1] -> Deco_3a8/2
  [m2] -> Deco_3a8/3
  [mux] -> Multiport Switch1/1
  [mux] -> Multiport Switch/1
  [mux] -> Multiport Switch2/1
  [mux] -> Multiport Switch3/1
  [ctrl_in] -> Switch5/1
  [ctrl_in] -> Switch4/1
  [ctrl_in] -> Switch3/1
  [ctrl_in] -> Switch2/1
  [ctrl_in] -> Switch1/1
  [ctrl_in] -> Switch/1
  data_in/1 -> [data_in]
  [data_in] -> Hc_12S-B80/1
  [data_in] -> Hc_12L-B360/1
  [data_in] -> Hc_23S-B60/1
  [data_in] -> Hc_23L-B270/1
  [data_in] -> Hc_56S-B48/1
  [data_in] -> Hc_56L-B216/1
  Hc_12S-B80/1 -> [d0]
  Hc_12L-B360/1 -> [d1]
  Hc_23S-B60/1 -> [d2]
  Hc_23L-B270/1 -> [d3]
  Hc_56S-B48/1 -> [d4]
  Hc_56L-B216/1 -> [d5]
  [d0] -> Multiport Switch1/2
  [d1] -> Multiport Switch1/3
  [d2] -> Multiport Switch1/4
  [d3] -> Multiport Switch1/5
  [d4] -> Multiport Switch1/6
  [d5] -> Multiport Switch1/7
  [n5] -> Multiport Switch4/7
  [n1] -> Multiport Switch4/3
  [n4] -> Multiport Switch4/6
  [n2] -> Multiport Switch4/4
  [mux] -> Multiport Switch4/1
  [n0] -> Multiport Switch4/2
  [n3] -> Multiport Switch4/5
  Multiport Switch4/1 -> next_frame/1
  Ground10/1 -> Multiport Switch4/8
  ctrl_in/1 -> [ctrl_in]
  gnd_ctrl1/1 -> Switch4/3
  gnd_ctrl2/1 -> Switch5/3
  gnd_ctrl3/1 -> Switch2/3
  gnd_ctrl4/1 -> Switch1/3
  gnd_ctrl5/1 -> Switch/3

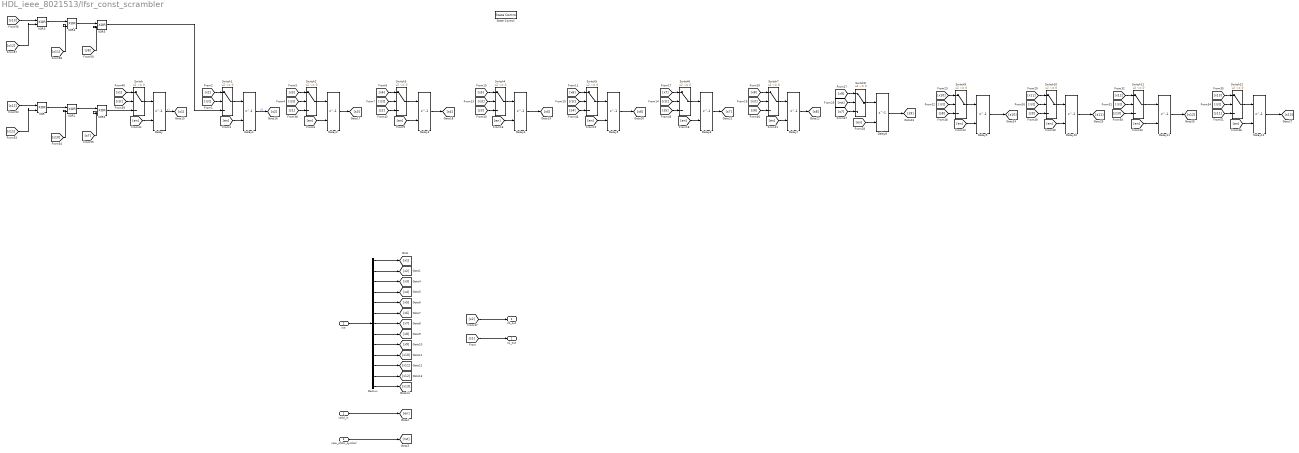
== system HDL_ieee_8021513/lfsr_const_scrambler ==
  valid_in : Inport
  init : Inport  Port=2
  new_ofdm_symbol : Inport  Port=3
  Delay{,1..12} (13 alike) : Delay  DelayLength=1  InitialCondition=0  ShowEnablePort=on  UseCircularBuffer=on
      settings: InputPortMap=u0,e6
  Demux : Demux  Outputs=13
  State Control : StateControl  StateControl=Synchronous
  Switch{,1..12} (13 alike) : Switch  Criteria=u2 ~= 0  SaturateOnIntegerOverflow=off  InputSameDT=off
  XOR{,1..5} (6 alike) : Logic  Operator=XOR  IconShape=distinctive  AllPortsSameDT=off  OutDataTypeStr=boolean
  s1_out : Outport  VectorParamsAs1DForOutWhenUnconnected=off
  s2_out : Outport  Port=2  VectorParamsAs1DForOutWhenUnconnected=off
  wires:
  [x13] -> Switch12/1
  Switch10/1 -> Delay10/1
  [x8] -> Switch7/1
  [rst] -> Switch10/2
  Switch3/1 -> Delay3/1
  Demux/6 -> [x6]
  Demux/12 -> [x12]
  Demux/1 -> [x1]
  Demux/8 -> [x8]
  [rst] -> Switch4/2
  Demux/7 -> [x7]
  Demux/3 -> [x3]
  Switch2/1 -> Delay2/1
  [en] -> Delay9/2
  [rst] -> Switch8/2
  [x12] -> Switch11/1
  [rst] -> Switch1/2
  [en] -> Delay12/2
  [rst] -> Switch3/2
  new_ofdm_symbol/1 -> [rst]
  Demux/9 -> [x9]
  [x1] -> Switch/1
  [x11] -> Switch10/1
  [x6] -> Switch5/1
  [rst] -> Switch5/2
  Switch4/1 -> Delay4/1
  Switch/1 -> Delay/1
  Demux/11 -> [x11]
  [rst] -> Switch7/2
  [x10] -> Switch9/1
  [rst] -> Switch12/2
  Switch5/1 -> Delay5/1
  [en] -> Delay5/2
  valid_in/1 -> [en]
  Demux/2 -> [x2]
  [en] -> Delay/2
  [x3] -> Switch2/1
  Demux/4 -> [x4]
  [en] -> Delay1/2
  [en] -> Delay2/2
  [rst] -> Switch6/2
  Switch11/1 -> Delay11/1
  [x7] -> Switch6/1
  Switch1/1 -> Delay1/1
  Switch9/1 -> Delay9/1
  [en] -> Delay11/2
  Demux/10 -> [x10]
  [en] -> Delay4/2
  [rst] -> Switch11/2
  Switch7/1 -> Delay7/1
  [en] -> Delay3/2
  init/1 -> Demux/1
  [en] -> Delay6/2
  Switch12/1 -> Delay12/1
  [x4] -> Switch3/1
  Switch8/1 -> Delay8/1
  [rst] -> Switch/2
  [x2] -> Switch1/1
  [x9] -> Switch8/1
  [en] -> Delay7/2
  Switch6/1 -> Delay6/1
  [en] -> Delay8/2
  Demux/13 -> [x13]
  [x5] -> Switch4/1
  [rst] -> Switch9/2
  [rst] -> Switch2/2
  Demux/5 -> [x5]
  [en] -> Delay10/2
  Delay/1 -> [s1]  "s1"
  [s1] -> s1_out/1
  Delay1/1 -> [s2]  "s2"
  Delay2/1 -> [s3]
  Delay3/1 -> [s4]
  Delay4/1 -> [s5]
  Delay5/1 -> [s6]
  Delay6/1 -> [s7]
  Delay7/1 -> [s8]
  Delay8/1 -> [s9]
  Delay9/1 -> [s10]
  Delay10/1 -> [s11]
  Delay11/1 -> [s12]
  Delay12/1 -> [s13]
  [s2] -> s2_out/1
  [s1] -> Switch2/3
  [s2] -> Switch3/3
  [s3] -> Switch4/3
  [s4] -> Switch5/3
  [s5] -> Switch6/3
  [s6] -> Switch7/3
  [s7] -> Switch8/3
  [s8] -> Switch9/3
  [s9] -> Switch10/3
  [s10] -> Switch11/3
  [s11] -> Switch12/3
  XOR1/1 -> XOR2/1
  XOR/1 -> XOR1/1
  [s12] -> XOR/1
  [s11] -> XOR/2
  [s10] -> XOR1/2
  [s7] -> XOR2/2
  [s13] -> XOR3/1
  XOR4/1 -> XOR5/1
  [s8] -> XOR5/2
  XOR3/1 -> XOR4/1
  [s11] -> XOR4/2
  [s12] -> XOR3/2
  XOR2/1 -> Switch/3
  XOR5/1 -> Switch1/3

== system HDL_ieee_8021513/next_frame_to_ready ==
  note: Given a next frame rising edge, this subsystem will generate a "ready" signal for the duration of "payloadWordsPerBlock0" clock cycles
  next_frame : Inport
  HDL Counter : hdlsllib/Sources/HDL Counter  CountType=Count limited  CountInit=0  CountStep=1  CountMax=CONST.payloadWordsPerBlock0-1  CountFromType=Initial value  CountFrom=0  CountResetPort=off  CountLoadPort=off  CountEnbPort=on  CountDirPort=off  CountHitOutputPort=on  CountDataType=Unsigned  CountWordLen=nextpow2(CONST.payloadWordsPerBlock0)  CountFracLen=0  CountSampTime=1
  Logical Operator2 : Logic  Operator=NOT  IconShape=distinctive  AllPortsSameDT=off  OutDataTypeStr=boolean
  Logical Operator3 : Logic  Operator=OR  IconShape=distinctive  AllPortsSameDT=off  OutDataTypeStr=boolean
  State Control : StateControl  StateControl=Synchronous
  Terminator : Terminator
  Unit Delay Enabled Synchronous : hdlsllib/Discrete/Unit Delay Enabled Synchronous  InitialCondition=0.0  SampleTime=-1
  rising_edge_detector : $bdroot/rising_edge_detector  SystemSampleTime=-1  VariantActivationTime=update diagram  AllowFlexibleInterface=on  Latency=0  AutoFrameSizeCalculation=off
  ready : Outport  VectorParamsAs1DForOutWhenUnconnected=off
  wires:
  next_frame/1 -> rising_edge_detector/1
  HDL Counter/2 -> Logical Operator2/1, Logical Operator3/2
  Logical Operator3/1 -> Unit Delay Enabled Synchronous/2
  Unit Delay Enabled Synchronous/1 -> ready/1, HDL Counter/1
  HDL Counter/1 -> Terminator/1
  Logical Operator2/1 -> Unit Delay Enabled Synchronous/1
  rising_edge_detector/1 -> Logical Operator3/1

== system HDL_ieee_8021513/ofdm_demod ==
  data_in : Inport
  valid_in : Inport  Port=2
  cp_len : Inport  Port=3
  reset : Inport  Port=4
  Constant2 : Constant  Value=CONST.N  OutDataTypeStr=fixdt(0,9,0)  SampleTime=-1  LockScale=on
  Constant3 : Constant  Value=length(CONST.rightGuard)  OutDataTypeStr=fixdt(0,6,0)  SampleTime=-1  LockScale=on
  Constant4 : Constant  Value=length(CONST.leftGuard)  OutDataTypeStr=fixdt(0,6,0)  SampleTime=-1  LockScale=on
  Data Type Conversion : DataTypeConversion  OutDataTypeStr=CONST.rxOFDMDemodDataType  SaturateOnIntegerOverflow=off  RndMeth=Floor
  Delay{,1..6} (7 alike) : Delay  DelayLength=1  InitialCondition=0  UseCircularBuffer=on
  OFDM Demodulator : whdlmod/OFDM Demodulator  OFDMParamsSource=Input port  MaxFFTLength=CONST.N  FFTLength=64  CPLength=16  NumLGsC=6  NumRGsC=5  CPFraction=off  CPFractionSource=Property  CPFractionValue=0.55  removeDCSubcarriers=off  enableResetInputPort=on  Normalize=off  RoundingMethod=Floor  SimulateUsing=Code generation
  data_out : Outport
  valid_out : Outport  Port=2
  ready : Outport  Port=3  VectorParamsAs1DForOutWhenUnconnected=off
  wires:
  Delay6/1 -> OFDM Demodulator/7
  Delay5/1 -> OFDM Demodulator/4
  Delay4/1 -> OFDM Demodulator/2
  Delay3/1 -> OFDM Demodulator/1
  Delay2/1 -> ready/1
  Delay1/1 -> valid_out/1
  Delay/1 -> Data Type Conversion/1
  Data Type Conversion/1 -> data_out/1
  reset/1 -> Delay6/1
  Constant2/1 -> OFDM Demodulator/3
  Constant3/1 -> OFDM Demodulator/6
  Constant4/1 -> OFDM Demodulator/5
  data_in/1 -> Delay3/1
  valid_in/1 -> Delay4/1
  cp_len/1 -> Delay5/1
  OFDM Demodulator/2 -> Delay1/1
  OFDM Demodulator/1 -> Delay/1
  OFDM Demodulator/3 -> Delay2/1

== system HDL_ieee_8021513/ofdm_modulator ==
  data_in : Inport
  valid_in : Inport  Port=2
  cp_len : Inport  Port=3
  rst : Inport  Port=4
  Constant2 : Constant  Value=CONST.N  OutDataTypeStr=fixdt(0,9,0)  SampleTime=-1  LockScale=on
  Constant3 : Constant  Value=length(CONST.rightGuard)  OutDataTypeStr=fixdt(0,6,0)  SampleTime=-1  LockScale=on
  Constant4 : Constant  Value=length(CONST.leftGuard)  OutDataTypeStr=fixdt(0,6,0)  SampleTime=-1  LockScale=on
  Delay{1..2,8..9,12} (5 alike) : Delay  DelayLength=1  InitialCondition=0  UseCircularBuffer=on
  Delay11 : Delay  InitialCondition=0  UseCircularBuffer=on
  Delay7 : Delay  InitialCondition=0  UseCircularBuffer=on
  OFDM Modulator : whdlmod/OFDM Modulator  OFDMParametersSource=Input Port  FFTLength=64  MaxFFTLength=CONST.N  CPLength=16  numLgSc=6  numRgSc=5  InsertDCNull=off  Windowing=off  WindowLength=4  MaxWindowLength=8  ResetInputPort=on  Normalize=on  RoundingMethod=Floor  SimulateUsing=Code generation
  State Control : StateControl  StateControl=Synchronous
  data_out : Outport
  valid_out : Outport  Port=2
  ready : Outport  Port=3  VectorParamsAs1DForOutWhenUnconnected=off
  wires:
  Delay2/1 -> OFDM Modulator/7
  rst/1 -> Delay2/1
  Delay12/1 -> ready/1  "ready_out"
  Delay11/1 -> valid_out/1
  Delay7/1 -> data_out/1
  Delay9/1 -> OFDM Modulator/4
  Delay1/1 -> OFDM Modulator/2
  Delay8/1 -> OFDM Modulator/1
  OFDM Modulator/3 -> Delay12/1
  OFDM Modulator/1 -> Delay7/1
  OFDM Modulator/2 -> Delay11/1
  Constant2/1 -> OFDM Modulator/3
  Constant3/1 -> OFDM Modulator/6
  Constant4/1 -> OFDM Modulator/5
  cp_len/1 -> Delay9/1
  data_in/1 -> Delay8/1
  valid_in/1 -> Delay1/1
